simulink model "QEI_Pulling"  (R2024b)
settings: Solver=FixedStepAuto  StartTime=0.0  StopTime=inf  FixedStep=0.001  RelTol=1e-3  EnableMultiTasking=on
libraries: stm32f4xxblockslib x5, stm32g4xxblockslib x3
settings Model: STM32="{\"EncoderBlockForG4\":[{\"ID\":\"QEI_Pulling:79\"},{\"ID\":\"QEI_Pulling:112\"},{\"ID\":\"QEI_Pulling:121\"}],\"DigitalPortRead\":[{\"ID\":\"QEI_Pulling:105\"},{\"ID\":\"QEI_Pulling:107\"},{\"ID\":\"QEI_Pulling:116\"},{\"ID\":\"QEI_Pulling:125\"},{\"ID\":\"QEI_Pulling:126\"}]}"  SimulationMode=external  Creator=spwkp  LastModifiedBy=spwkp
settings OptimizationCC: DefaultParameterBehavior=Inlined  EnhancedBackFolding=on  PassReuseOutputArgsAs=Individual arguments  ZeroExternalMemoryAtStartup=off  ZeroInternalMemoryAtStartup=off  MaxStackSize=512  OptimizeBlockOrder=speed  DifferentSizesBufferReuse=on  OptimizationCustomize=off  EfficientTunableParamExpr=on
settings DebuggingCC: ParameterTunabilityLossMsg=error
settings HardwareCC: ProdBitPerPointer=32  ProdBitPerSizeT=32  ProdBitPerPtrDiffT=32  ProdLargestAtomicInteger=Long  ProdLargestAtomicFloat=Double  ProdWordSize=32  ProdLongLongMode=on  ProdHWDeviceType=ARM Compatible->ARM Cortex-M
settings SFSimCC: MATLABDynamicMemAlloc=off
settings RTWCC: Description=Embedded Coder  SystemTargetFile=ert.tlc  HardwareBoard=STM32G4xx Based  TemplateMakefile=ert_default_tmf  Toolchain=GNU Tools for ARM Embedded Processors
settings CodeAppCC: ForceParamTrailComments=on  IgnoreCustomStorageClasses=off  OperatorAnnotations=on  SimulinkDataObjDesc=on  SFDataObjDesc=on  InsertBlockDesc=on
settings ERTTargetCC: TargetLangStandard=C99 (ISO)  CodeReplacementLibrary=ARM Cortex-M  ExtModeTransport=3  ExtModeStaticAlloc=on  ExtModeStaticAllocSize=2048  ExtModeMexFile=ext_xcp  ExtModeIntrfLevel=Level2 - Open

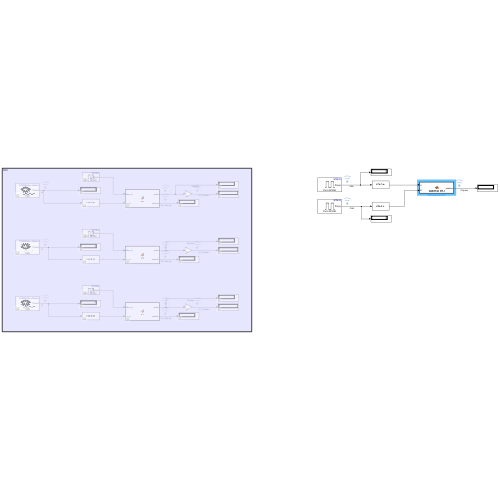
[thumbnail: Simulink's stored preview of the top-level diagram]
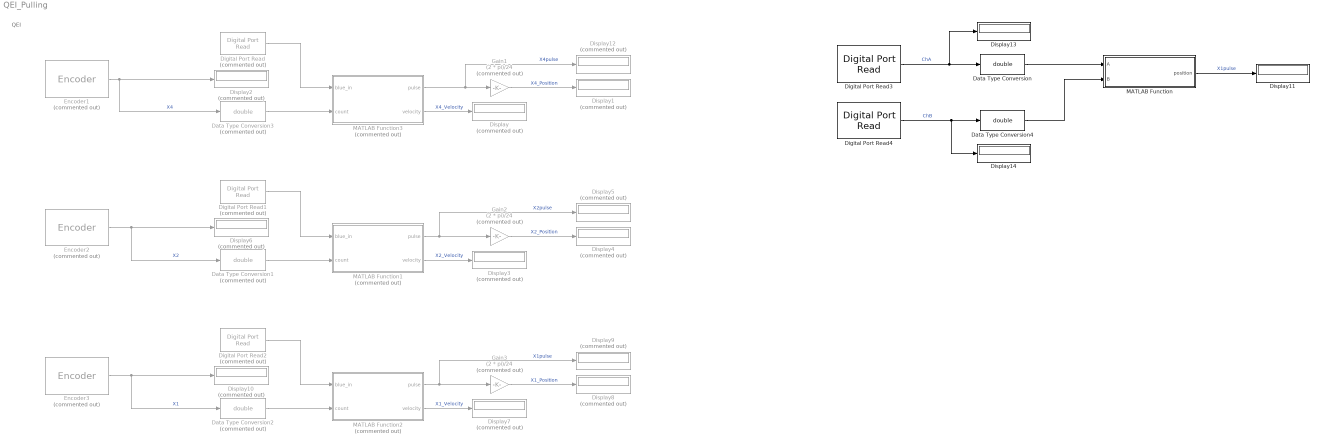
== system QEI_Pulling ==
  note: QEI
  Data Type Conversion : DataTypeConversion  OutDataTypeStr=double  SaturateOnIntegerOverflow=off  RndMeth=Floor
  Data Type Conversion1 : DataTypeConversion  Commented=on  OutDataTypeStr=double  SaturateOnIntegerOverflow=off  RndMeth=Floor
  Data Type Conversion2 : DataTypeConversion  Commented=on  OutDataTypeStr=double  SaturateOnIntegerOverflow=off  RndMeth=Floor
  Data Type Conversion3 : DataTypeConversion  Commented=on  OutDataTypeStr=double  SaturateOnIntegerOverflow=off  RndMeth=Floor
  Data Type Conversion4 : DataTypeConversion  OutDataTypeStr=double  SaturateOnIntegerOverflow=off  RndMeth=Floor
  Digital Port Read : stm32f4xxblockslib/Digital Port Read  Commented=on  PortName=GPIOC  PinNumber=[13]  ReadOperation=on  IOAsArray=on  SampleTime=-1  EnableSimPort=off  hoistedMaskSrc=ECSoC/ECSimCodegen/Digital Port Read
      settings: LibrarySourceBlock=stm32g4xxblockslib/Digital Port Read
  Digital Port Read1 : stm32f4xxblockslib/Digital Port Read  Commented=on  PortName=GPIOC  PinNumber=[13]  ReadOperation=on  IOAsArray=on  SampleTime=-1  EnableSimPort=off  hoistedMaskSrc=ECSoC/ECSimCodegen/Digital Port Read
      settings: LibrarySourceBlock=stm32g4xxblockslib/Digital Port Read
  Digital Port Read2 : stm32f4xxblockslib/Digital Port Read  Commented=on  PortName=GPIOC  PinNumber=[13]  ReadOperation=on  IOAsArray=on  SampleTime=-1  EnableSimPort=off  hoistedMaskSrc=ECSoC/ECSimCodegen/Digital Port Read
      settings: LibrarySourceBlock=stm32g4xxblockslib/Digital Port Read
  Digital Port Read3 : stm32f4xxblockslib/Digital Port Read  PortName=GPIOB  PinNumber=[13]  ReadOperation=on  IOAsArray=on  SampleTime=-1  EnableSimPort=off  hoistedMaskSrc=ECSoC/ECSimCodegen/Digital Port Read
      settings: LibrarySourceBlock=stm32g4xxblockslib/Digital Port Read
  Digital Port Read4 : stm32f4xxblockslib/Digital Port Read  PortName=GPIOB  PinNumber=[14]  ReadOperation=on  IOAsArray=on  SampleTime=-1  EnableSimPort=off  hoistedMaskSrc=ECSoC/ECSimCodegen/Digital Port Read
      settings: LibrarySourceBlock=stm32g4xxblockslib/Digital Port Read
  Display{,1..10,12} (12 alike) : Display  Commented=on
      Display1 settings: Format=decimal (Stored Integer)
      Display4 settings: Format=decimal (Stored Integer)
      Display8 settings: Format=decimal (Stored Integer)
  Display11 : Display
  Display13 : Display
  Display14 : Display
  Encoder1 : stm32g4xxblockslib/Encoder  Commented=on  TimerModule=TIM3  EnableResetInput=off  OutputCountAfterFirstIndex=off  OutputValidIndex=off  OutputDirection=off  OutputStatus=off  SampleTime=-1
  Encoder2 : stm32g4xxblockslib/Encoder  Commented=on  TimerModule=TIM4  EnableResetInput=off  OutputCountAfterFirstIndex=off  OutputValidIndex=off  OutputDirection=off  OutputStatus=off  SampleTime=-1
  Encoder3 : stm32g4xxblockslib/Encoder  Commented=on  TimerModule=TIM8  EnableResetInput=off  OutputCountAfterFirstIndex=off  OutputValidIndex=off  OutputDirection=off  OutputStatus=off  SampleTime=-1
  Gain1 : Gain  Commented=on  Gain=(2 * pi)/24
  Gain2 : Gain  Commented=on  Gain=(2 * pi)/24
  Gain3 : Gain  Commented=on  Gain=(2 * pi)/24
  MATLAB Function : MATLAB Function  TreatAsAtomicUnit=on
  MATLAB Function1 : MATLAB Function  Commented=on  TreatAsAtomicUnit=on
  MATLAB Function2 : MATLAB Function  Commented=on  TreatAsAtomicUnit=on
  MATLAB Function3 : MATLAB Function  Commented=on  TreatAsAtomicUnit=on
  wires:
  Encoder1/1 -> Data Type Conversion3/1, Display2/1  "X4"
  Gain1/1 -> Display1/1  "X4_Position"
  MATLAB Function3/1(pulse) -> Gain1/1, Display12/1  "X4pulse"
  MATLAB Function3/2(velocity) -> Display/1  "X4_Velocity"
  Data Type Conversion3/1 -> MATLAB Function3/2(count)
  Digital Port Read/1 -> MATLAB Function3/1(blue_in)
  Digital Port Read1/1 -> MATLAB Function1/1(blue_in)
  MATLAB Function1/2(velocity) -> Display3/1  "X2_Velocity"
  Data Type Conversion1/1 -> MATLAB Function1/2(count)
  Gain2/1 -> Display4/1  "X2_Position"
  MATLAB Function1/1(pulse) -> Gain2/1, Display5/1  "X2pulse"
  Encoder2/1 -> Data Type Conversion1/1, Display6/1  "X2"
  Digital Port Read2/1 -> MATLAB Function2/1(blue_in)
  MATLAB Function2/2(velocity) -> Display7/1  "X1_Velocity"
  Data Type Conversion2/1 -> MATLAB Function2/2(count)
  Gain3/1 -> Display8/1  "X1_Position"
  MATLAB Function2/1(pulse) -> Gain3/1, Display9/1  "X1pulse"
  Encoder3/1 -> Data Type Conversion2/1, Display10/1  "X1"
  Digital Port Read4/1 -> Display14/1, Data Type Conversion4/1  "ChB"
  Digital Port Read3/1 -> Display13/1, Data Type Conversion/1  "ChA"
  Data Type Conversion/1 -> MATLAB Function/1(A)
  MATLAB Function/1(position) -> Display11/1  "X1pulse"
  Data Type Conversion4/1 -> MATLAB Function/2(B)

== matlab function QEI_Pulling/MATLAB Function1 ==
  data: blue_in input; count input double size=[1 1]; pulse output double size=[1 1 ]; velocity output
function [pulse, velocity] = X2(blue_in, count)
    %#codegen
    
    % ประกาศตัวแปร persistent เพื่อเก็บค่าตัวนับก่อนหน้าและตำแหน่งที่คลายห่อก่อนหน้า
    persistent previousCount unwrappedPositionPrev;
    
    % กำหนดค่าเริ่มต้นให้ตัวแปร persistent เมื่อเรียกใช้งานครั้งแรก
    if isempty(previousCount)
        previousCount = count;
        unwrappedPositionPrev = 0;  % กำหนดตำแหน่งคลายห่อเริ่มต้นเป็นศูนย์
    end

    % กำหนดขอบเขตของ encoder
    encoderMax = 65520;   % ค่าสูงสุดสำหรับ encoder แบบ 16-bit (0-65535)
    threshold = encoderMax / 2;  % ค่า threshold สำหรับตรวจจับ overflow หรือ underflow

    % คำนวณค่าความแตกต่างระหว่างค่าปัจจุบันกับค่าก่อนหน้า
    diff_count = count - previousCount;

    % คำนวณความเร็วเชิงมุม (Angular Velocity)
    Ts = 0.01; % กำหนด Sampling Time (เช่น 10ms)
    PPR = 24; % จำนวนพัลส์ต่อรอบ
    velocity = ((diff_count / PPR) / Ts) * 60; % Velocity เป็น RPM

    % ตรวจจับการ overflow และ underflow
    if diff_count > threshold
        % พบการ overflow (เช่น count เปลี่ยนจาก 65535 กลับไปที่ 0)
        pulse = unwrappedPositionPrev + (diff_count - encoderMax);
    elseif diff_count < -threshold
        % พบการ underflow (เช่น count เปลี่ยนจาก 0 เป็น 65535)
        pulse = unwrappedPositionPrev + (diff_count + encoderMax);
    else
        % กรณีปกติที่ไม่มี overflow/underflow
        pulse = unwrappedPositionPrev + diff_count;
    end

    if blue_in == 1
        pulse = 0;
        velocity = 0;
    end
    % อัปเดตตัวแปร persistent เพื่อใช้ในรอบถัดไป
    previousCount = count;
    unwrappedPositionPrev = pulse; 
end

== matlab function QEI_Pulling/MATLAB Function3 ==
  data: blue_in input; count input double size=[1 1]; pulse output double size=[1 1 ]; velocity output
function [pulse, velocity] = X4(blue_in, count)
    %#codegen
    
    % ประกาศตัวแปร persistent เพื่อเก็บค่าตัวนับก่อนหน้าและตำแหน่งที่คลายห่อก่อนหน้า
    persistent previousCount unwrappedPositionPrev;
    
    % กำหนดค่าเริ่มต้นให้ตัวแปร persistent เมื่อเรียกใช้งานครั้งแรก
    if isempty(previousCount)
        previousCount = count;
        unwrappedPositionPrev = 0;  % กำหนดตำแหน่งคลายห่อเริ่มต้นเป็นศูนย์
    end

    % กำหนดขอบเขตของ encoder
    encoderMax = 65520;   % ค่าสูงสุดสำหรับ encoder แบบ 16-bit (0-65535)
    threshold = encoderMax / 2;  % ค่า threshold สำหรับตรวจจับ overflow หรือ underflow

    % คำนวณค่าความแตกต่างระหว่างค่าปัจจุบันกับค่าก่อนหน้า
    diff_count = count - previousCount;

    % คำนวณความเร็วเชิงมุม (Angular Velocity)
    Ts = 0.01; % กำหนด Sampling Time (เช่น 10ms)
    PPR = 24; % จำนวนพัลส์ต่อรอบ
    velocity = ((diff_count / PPR) / Ts) * 60; % Velocity เป็น RPM

    % ตรวจจับการ overflow และ underflow
    if diff_count > threshold
        % พบการ overflow (เช่น count เปลี่ยนจาก 65535 กลับไปที่ 0)
        pulse = unwrappedPositionPrev + (diff_count - encoderMax);
    elseif diff_count < -threshold
        % พบการ underflow (เช่น count เปลี่ยนจาก 0 เป็น 65535)
        pulse = unwrappedPositionPrev + (diff_count + encoderMax);
    else
        % กรณีปกติที่ไม่มี overflow/underflow
        pulse = unwrappedPositionPrev + diff_count;
    end

    if blue_in == 1
        pulse = 0;
        velocity = 0;
    end
    % อัปเดตตัวแปร persistent เพื่อใช้ในรอบถัดไป
    previousCount = count;
    unwrappedPositionPrev = pulse; 
end

== matlab function QEI_Pulling/MATLAB Function2 ==
  data: blue_in input; count input double size=[1 1]; pulse output double size=[1 1 ]; velocity output
function [pulse, velocity] = X1(blue_in, count)
    %#codegen
    
    % ประกาศตัวแปร persistent เพื่อเก็บค่าตัวนับก่อนหน้าและตำแหน่งที่คลายห่อก่อนหน้า
    persistent previousCount unwrappedPositionPrev;
    
    % กำหนดค่าเริ่มต้นให้ตัวแปร persistent เมื่อเรียกใช้งานครั้งแรก
    if isempty(previousCount)
        previousCount = count;
        unwrappedPositionPrev = 0;  % กำหนดตำแหน่งคลายห่อเริ่มต้นเป็นศูนย์
    end

    % กำหนดขอบเขตของ encoder
    encoderMax = 65520;   % ค่าสูงสุดสำหรับ encoder แบบ 16-bit (0-65535)
    threshold = encoderMax / 2;  % ค่า threshold สำหรับตรวจจับ overflow หรือ underflow

    % คำนวณค่าความแตกต่างระหว่างค่าปัจจุบันกับค่าก่อนหน้า
    diff_count = count - previousCount;

    % คำนวณความเร็วเชิงมุม (Angular Velocity)
    Ts = 0.01; % กำหนด Sampling Time (เช่น 10ms)
    PPR = 24; % จำนวนพัลส์ต่อรอบ
    velocity = ((diff_count / PPR) / Ts) * 60; % Velocity เป็น RPM

    % ตรวจจับการ overflow และ underflow
    if diff_count > threshold
        % พบการ overflow (เช่น count เปลี่ยนจาก 65535 กลับไปที่ 0)
        pulse = unwrappedPositionPrev + (diff_count - encoderMax);
    elseif diff_count < -threshold
        % พบการ underflow (เช่น count เปลี่ยนจาก 0 เป็น 65535)
        pulse = unwrappedPositionPrev + (diff_count + encoderMax);
    else
        % กรณีปกติที่ไม่มี overflow/underflow
        pulse = unwrappedPositionPrev + diff_count;
    end

    if blue_in == 1
        pulse = 0;
        velocity = 0;
    end
    % อัปเดตตัวแปร persistent เพื่อใช้ในรอบถัดไป
    previousCount = count;
    unwrappedPositionPrev = pulse; 
end

== matlab function QEI_Pulling/MATLAB Function ==
  data: A input; position output; B input
function position = readEncoderX1(A, B)
    % readEncoderX1 - Read encoder position using X1 mode with polling
    % A and B are the input signals from the encoder channels A and B
    % position returns the current encoder position, counting forward and backward
    
    persistent lastA count;
    if isempty(lastA) || isempty(count)
        % Initialize variables if not set
        lastA = 0;
        count = 0;
    end
    
    % Read current states of A and B
    currentA = A;  % Replace with the actual read function for channel A
    currentB = B;  % Replace with the actual read function for channel B
    
    % Check for rising edge of A (from 0 to 1)
    if lastA == 0 && currentA == 1
        % Determine direction based on the state of B
        if currentB == 0
            count = count + 1;  % Forward count
        else
            count = count - 1;  % Backward count
        end
    end
    
    % Update last value of A for the next polling cycle
    lastA = currentA;
    
    % Return the current position count
    position = count;
end
